simulink model "Bebop5_like3_but_dist_toward_end"  (R2018a)
settings: Solver=VariableStepAuto  StartTime=0.0  StopTime=50  FixedStep=.04  MaxStep=1.00  MinStep=0.005  RelTol=10  AbsTol=10
values from neighbouring files (symbols this model uses):
  flightplan = [dist,0,height,deg2rad(090) ... (first row only)    [compare_cubic_spline_1.m]    (also in initialize_race_realtime.m; initialize_race_realtime_backup_cubic.m; plot_sim.m = [ 4.348, -0.278, height, deg2rad(  0); test_b_spline.m)
  FOV = 1.05    [initialize_race_realtime.m]    (also in initialize_race_realtime_backup_cubic.m)
  g = 9.81    [initialize_race_no_realtime.m]    (also in initialize_race_realtime.m; initialize_race_realtime_backup_cubic.m; moving_average_rls_own.m = P(i-1)*meas*(lambda+meas*P(i-1)*meas)^-1)
  gate_size = 1.4    [initialize_race_realtime.m]    (also in initialize_race_realtime_backup_cubic.m)
  gates = sim_gates(:,:,1)    [eval_sim.m]    (also in initialize_race_realtime.m = [dist,0,height,deg2rad(110); initialize_race_realtime_backup_cubic.m = [dist,0,height,deg2rad(110); plot_sim.m)
  I = [1 0 0 ... (first row only)    [Bebop_sim_init.m]    (also in initialize_race_no_realtime.m; initialize_race_realtime.m; initialize_race_realtime_backup_cubic.m; moving_averge_rls_download.m = ones(1,N))
  init_std_dev = [1.0*ones(1,3),deg2rad(30)]    [initialize_race_realtime.m]    (also in initialize_race_realtime_backup_cubic.m)
  m = 0.68    [calc_plot_spline.m]    (also in calc_spline.m; compare_cubic_spline_1.m = vpasolve(e,r); compare_cubic_spline_2.m = r/3*(-sin(dp)+sqrt(sin(dp)^2-6*cos(dp)+6)); initialize_race_no_realtime.m = 2)
  max_rot_Z = (90)*pi/180    (= 1.57079632679)    [Bebop_sim_init.m]    (also in initialize_race_no_realtime.m = 1.0471975512; initialize_race_realtime.m; initialize_race_realtime_backup_cubic.m; run_batch1.m = list_agility(idx_agility)*max_rot_Z)
  max_theta_X = (40)*pi/180    (= 0.698131700798)    [Bebop_sim_init.m]    (also in initialize_race_no_realtime.m = 0.13962634016; initialize_race_realtime.m = 1.308996939; initialize_race_realtime_backup_cubic.m = 1.308996939; run_batch1.m = list_agility(idx_agility)*max_theta_X)
  max_theta_Y = (40)*pi/180    (= 0.698131700798)    [Bebop_sim_init.m]    (also in initialize_race_no_realtime.m = 0.13962634016; initialize_race_realtime.m = 1.308996939; initialize_race_realtime_backup_cubic.m = 1.308996939; run_batch1.m = list_agility(idx_agility)*max_theta_Y)
  max_v_Z = .5    (= 0.5)    [Bebop_sim_init.m]    (also in initialize_race_no_realtime.m = 1; initialize_race_realtime.m = 3; initialize_race_realtime_backup_cubic.m = 3; run_batch1.m = list_agility(idx_agility)*max_v_Z)
  max_vel = 1.5    [initialize_race_realtime.m]    (also in initialize_race_realtime_backup_cubic.m; run_batch1.m = list_speed(idx_speed); run_batch2.m = list_speed(idx_speed); run_batch3.m = list_speed(idx_speed))
  std_dev_factor = 1.0    (= 1)    [initialize_race_realtime.m]
  std_dev_switch = std_dev_factor/5    (= 0.2)    [initialize_race_realtime.m]
undefined symbols (not defined in the file or in its folder): fspecial, gray, Rec, SDTV
libraries: simulink x11, sharedtransform x11, visionanalysis x7, visiontextngfix x5, visiontransforms x3, aerolibactuator x2, aerolibutil x2, vrlib x2, visionstatistics x2, visionconversions x2, shared6dof x1, visionsinks x1
(part 3 of 4)

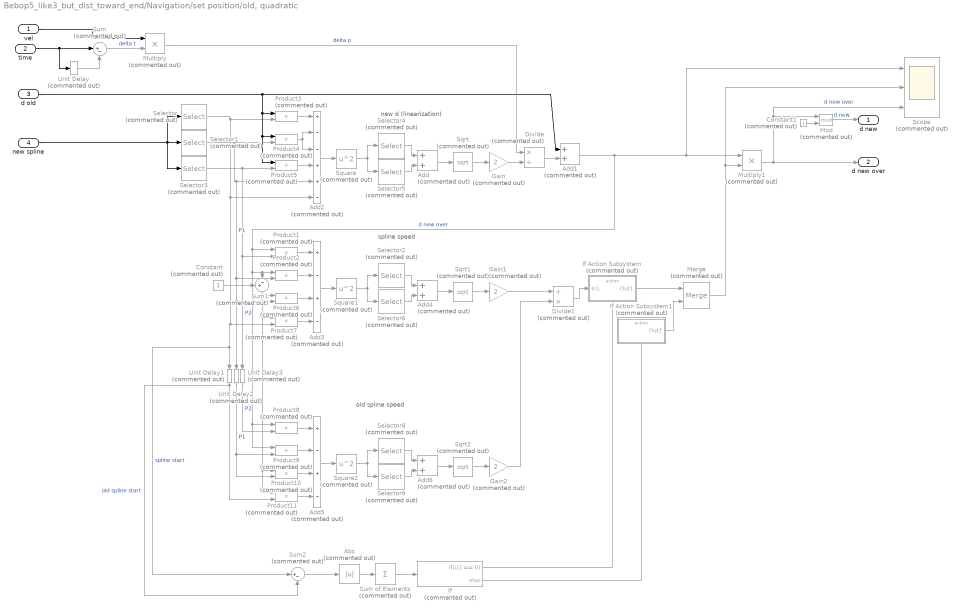
== system Bebop5_like3_but_dist_toward_end/Navigation/set position/old, quadratic ==
  note: old spline speed
  note: spline speed
  note: new d (linearization)
  vel : Inport
  time : Inport  Port=2
  d old : Inport  Port=3
  new spline : Inport  Port=4
  Abs : Abs  Commented=on
  Add{,1,4,6} (4 alike) : Sum  Commented=on
  Add2 : Sum  Commented=on  Inputs=+--++-
  Add3 : Sum  Commented=on  Inputs=+-+-
  Add5 : Sum  Commented=on  Inputs=+-+-
  Constant : Constant  Commented=on
  Constant1 : Constant  Commented=on
  Divide : Product  Commented=on  Inputs=*/
  Divide1 : Product  Commented=on  Inputs=/*
  Gain : Gain  Commented=on  Gain=2
  Gain1 : Gain  Commented=on  Gain=2
  Gain2 : Gain  Commented=on  Gain=2
  If : If  Commented=on  IfExpression=u1 == 0
  If Action Subsystem : Subsystem  Commented=on  TreatAsAtomicUnit=on
  If Action Subsystem1 : Subsystem  Commented=on  TreatAsAtomicUnit=on
  Merge : Merge  Commented=on
  Mod : Math  Commented=on  Operator=mod  SaturateOnIntegerOverflow=on
  Multiply : Product  Commented=on
  Multiply1 : Product  Commented=on
  Product{1..11} (11 alike) : Product  Commented=on
  Scope : Scope  Commented=on  NumInputPorts=3
  Selector : Selector  Commented=on  NumberOfDimensions=2  IndexMode=Zero-based  InputPortWidth=3  IndexOptions=Index vector (dialog),Index vector (dialog)  Indices=0,[0 1 2]  OutputSizes=1,1
  Selector1 : Selector  Commented=on  NumberOfDimensions=2  IndexMode=Zero-based  InputPortWidth=3  IndexOptions=Index vector (dialog),Index vector (dialog)  Indices=1,[0 1 2]  OutputSizes=1,1
  Selector2 : Selector  Commented=on  IndexMode=Zero-based  InputPortWidth=3  IndexOptions=Index vector (dialog)  Indices=1  OutputSizes=1
  Selector3 : Selector  Commented=on  NumberOfDimensions=2  IndexMode=Zero-based  InputPortWidth=3  IndexOptions=Index vector (dialog),Index vector (dialog)  Indices=2,[0 1 2]  OutputSizes=1,1
  Selector4 : Selector  Commented=on  IndexMode=Zero-based  InputPortWidth=3  IndexOptions=Index vector (dialog)  Indices=1  OutputSizes=1
  Selector5 : Selector  Commented=on  IndexMode=Zero-based  InputPortWidth=3  IndexOptions=Index vector (dialog)  Indices=0  OutputSizes=1
  Selector6 : Selector  Commented=on  IndexMode=Zero-based  InputPortWidth=3  IndexOptions=Index vector (dialog)  Indices=0  OutputSizes=1
  Selector8 : Selector  Commented=on  IndexMode=Zero-based  InputPortWidth=3  IndexOptions=Index vector (dialog)  Indices=1  OutputSizes=1
  Selector9 : Selector  Commented=on  IndexMode=Zero-based  InputPortWidth=3  IndexOptions=Index vector (dialog)  Indices=0  OutputSizes=1
  Sqrt : Sqrt  Commented=on  SaturateOnIntegerOverflow=on
  Sqrt1 : Sqrt  Commented=on  SaturateOnIntegerOverflow=on
  Sqrt2 : Sqrt  Commented=on  SaturateOnIntegerOverflow=on
  Square : Math  Commented=on  Operator=square  SaturateOnIntegerOverflow=on
  Square1 : Math  Commented=on  Operator=square  SaturateOnIntegerOverflow=on
  Square2 : Math  Commented=on  Operator=square  SaturateOnIntegerOverflow=on
  Sum : Sum  Commented=on  Inputs=|+-
  Sum of Elements : Sum  Commented=on  Inputs=+
  Sum1 : Sum  Commented=on  Inputs=+-|
  Sum2 : Sum  Commented=on  Inputs=|+-
  Unit Delay{,1..3} (4 alike) : UnitDelay  Commented=on  SampleTime=-1
  d new : Outport
  d new over : Outport  Port=2
  wires:
  Product6/1 -> Add3/3
  Add5/1 -> Square2/1
  If Action Subsystem/1(Out1) -> Merge/1
  Gain/1 -> Divide/2
  Product10/1 -> Add5/3
  Add3/1 -> Square1/1
  Product11/1 -> Add5/4
  Product8/1 -> Add5/1
  Abs/1 -> Sum of Elements/1
  Sum2/1 -> Abs/1
  Gain1/1 -> Divide1/1
  Add4/1 -> Sqrt1/1
  Add1/1 -> Product1/1, Product8/1, Product9/1, Product2/1, Sum1/2, Scope/1, Multiply1/1  "d new over"
  Add/1 -> Sqrt/1
  Product5/1 -> Add2/4
  Selector/1 -> Product3/2, Add2/6, Unit Delay1/1, Sum2/1, Product7/2  "spline start"
  Constant/1 -> Sum1/1
  Sqrt2/1 -> Gain2/1
  Product4/1 -> Add2/2, Add2/3
  Square/1 -> Selector5/1, Selector4/1
  Product2/1 -> Add3/2
  Selector5/1 -> Add/2
  vel/1 -> Multiply/1
  Product3/1 -> Add2/1
  d old/1 -> Add1/1, Product3/1, Product4/1, Product5/1
  Add6/1 -> Sqrt2/1
  Sum1/1 -> Product11/1, Product10/1, Product7/1, Product6/1
  Unit Delay/1 -> Sum/2
  Divide/1 -> Add1/2
  Mod/1 -> d new/1  "d new"
  time/1 -> Unit Delay/1, Sum/1
  Merge/1 -> Scope/2, Multiply1/2
  If/1 -> If Action Subsystem/Action
  Square1/1 -> Selector2/1, Selector6/1
  Selector3/1 -> Product5/2, Unit Delay3/1, Product1/2  "P2"
  new spline/1 -> Selector/1, Selector3/1, Selector1/1
  Selector6/1 -> Add4/2
  Selector1/1 -> Product4/2, Add2/5, Product2/2, Unit Delay2/1, Product6/2  "P1"
  Multiply1/1 -> d new over/1, Scope/3, Mod/1  "d new over"
  Divide1/1 -> If Action Subsystem/1(In1)
  If/2 -> If Action Subsystem1/Action
  Sqrt/1 -> Gain/1
  Product1/1 -> Add3/1
  Unit Delay2/1 -> Product9/2, Product10/2  "P1"
  Add2/1 -> Square/1
  Unit Delay1/1 -> Product11/2, Sum2/2  "old spline start"
  Selector8/1 -> Add6/1
  Sum/1 -> Multiply/2  "delta t"
  Selector9/1 -> Add6/2
  If Action Subsystem1/1(Out1) -> Merge/2
  Sqrt1/1 -> Gain1/1
  Selector2/1 -> Add4/1
  Unit Delay3/1 -> Product8/2  "P2"
  Square2/1 -> Selector8/1, Selector9/1
  Multiply/1 -> Divide/1  "delta p"
  Constant1/1 -> Mod/2
  Product9/1 -> Add5/2
  Sum of Elements/1 -> If/1
  Product7/1 -> Add3/4
  Selector4/1 -> Add/1
  Gain2/1 -> Divide1/2

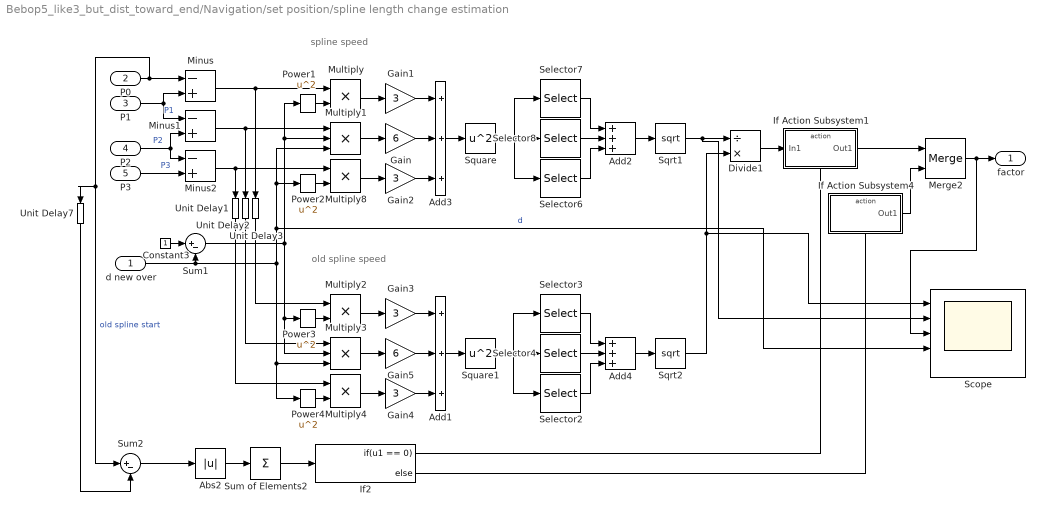
== system Bebop5_like3_but_dist_toward_end/Navigation/set position/spline length change estimation ==
  note: old spline speed
  note: spline speed
  d new over : Inport
  P0 : Inport  Port=2
  P1 : Inport  Port=3
  P2 : Inport  Port=4
  P3 : Inport  Port=5
  Abs2 : Abs
  Add{1..4} (4 alike) : Sum  Inputs=+++
  Constant3 : Constant
  Divide1 : Product  Inputs=/*
  Gain : Gain  Gain=6
  Gain{1..4} (4 alike) : Gain  Gain=3
  Gain5 : Gain  Gain=6
  If Action Subsystem1 : Subsystem  TreatAsAtomicUnit=on
  If Action Subsystem4 : Subsystem  TreatAsAtomicUnit=on
  If2 : If  IfExpression=u1 == 0
  Merge2 : Merge
  Minus : Sum  Inputs=-+
  Minus1 : Sum  Inputs=-+
  Minus2 : Sum  Inputs=-+
  Multiply{,2,4,8} (4 alike) : Product
  Multiply1 : Product  Inputs=3
  Multiply3 : Product  Inputs=3
  Power{1..4} (4 alike) : Math  Operator=square  SaturateOnIntegerOverflow=on
  Scope : Scope  NumInputPorts=5
  Selector2 : Selector  IndexMode=Zero-based  InputPortWidth=3  IndexOptions=Index vector (dialog)  Indices=2  OutputSizes=1
  Selector3 : Selector  IndexMode=Zero-based  InputPortWidth=3  IndexOptions=Index vector (dialog)  Indices=0  OutputSizes=1
  Selector4 : Selector  IndexMode=Zero-based  InputPortWidth=3  IndexOptions=Index vector (dialog)  Indices=1  OutputSizes=1
  Selector6 : Selector  IndexMode=Zero-based  InputPortWidth=3  IndexOptions=Index vector (dialog)  Indices=2  OutputSizes=1
  Selector7 : Selector  IndexMode=Zero-based  InputPortWidth=3  IndexOptions=Index vector (dialog)  Indices=0  OutputSizes=1
  Selector8 : Selector  IndexMode=Zero-based  InputPortWidth=3  IndexOptions=Index vector (dialog)  Indices=1  OutputSizes=1
  Sqrt1 : Sqrt  SaturateOnIntegerOverflow=on
  Sqrt2 : Sqrt  SaturateOnIntegerOverflow=on
  Square : Math  Operator=square  SaturateOnIntegerOverflow=on
  Square1 : Math  Operator=square  SaturateOnIntegerOverflow=on
  Sum of Elements2 : Sum  Inputs=+
  Sum1 : Sum  Inputs=|+-
  Sum2 : Sum  Inputs=|+-
  Unit Delay{1..3,7} (4 alike) : UnitDelay  SampleTime=-1
  factor : Outport
  wires:
  P2/1 -> Minus1/2, Minus2/1  "P2"
  Power1/1 -> Multiply/2
  Minus1/1 -> Unit Delay2/1, Multiply1/1
  Constant3/1 -> Sum1/1
  Minus/1 -> Unit Delay3/1, Multiply/1
  P1/1 -> Minus/2, Minus1/1  "P1"
  Multiply8/1 -> Gain2/1
  Power2/1 -> Multiply8/2
  Multiply/1 -> Gain1/1
  P3/1 -> Minus2/2  "P3"
  Minus2/1 -> Unit Delay1/1, Multiply8/1
  Multiply1/1 -> Gain/1
  Gain/1 -> Add3/2
  Power3/1 -> Multiply2/2
  Multiply2/1 -> Gain3/1
  Gain5/1 -> Add1/2
  Multiply4/1 -> Gain4/1
  Power4/1 -> Multiply4/2
  Multiply3/1 -> Gain5/1
  Unit Delay1/1 -> Multiply4/1
  d new over/1 -> Sum1/2, Power4/1, Multiply3/3, Scope/4, Multiply1/3, Power2/1  "d"
  Unit Delay3/1 -> Multiply2/1
  Unit Delay2/1 -> Multiply3/1
  Sum1/1 -> Multiply3/2, Power3/1, Power1/1, Multiply1/2
  Selector7/1 -> Add2/1
  Selector6/1 -> Add2/3
  Add2/1 -> Sqrt1/1
  Selector8/1 -> Add2/2
  Selector4/1 -> Add4/2
  Selector3/1 -> Add4/1
  Selector2/1 -> Add4/3
  Add4/1 -> Sqrt2/1
  Add3/1 -> Square/1
  Add1/1 -> Square1/1
  Abs2/1 -> Sum of Elements2/1
  Sum of Elements2/1 -> If2/1
  Sum2/1 -> Abs2/1
  Unit Delay7/1 -> Sum2/2
  P0/1 -> Sum2/1, Unit Delay7/1, Minus/1  "old spline start"
  If2/1 -> If Action Subsystem1/Action
  Sqrt2/1 -> Scope/1, Divide1/2
  Sqrt1/1 -> Scope/2, Divide1/1
  If2/2 -> If Action Subsystem4/Action
  If Action Subsystem1/1(Out1) -> Merge2/1
  Divide1/1 -> If Action Subsystem1/1(In1)
  If Action Subsystem4/1(Out1) -> Merge2/2
  Merge2/1 -> Scope/3, factor/1
  Gain1/1 -> Add3/1
  Gain2/1 -> Add3/3
  Gain3/1 -> Add1/1
  Gain4/1 -> Add1/3
  Square/1 -> Selector6/1, Selector7/1, Selector8/1
  Square1/1 -> Selector2/1, Selector3/1, Selector4/1

== system Bebop5_like3_but_dist_toward_end/Vision System/Harris corner detection/Harris Corners ==
  Threshold : Inport
  Corner Detection : visionanalysis/Corner Detection  method=Harris corner detection (Harris & Stephens)  factor=0.01  filter=fspecial('gaussian', [1 9], 3)  thrInten=0.1  thrAngle=157.5  output=Obsolete9b  outputInUse=Corner location  maxNum=5  thrMetric=0.01  neighborSize=[25 25]  isOutVarDim=on  accumMode=Binary point scaling  accumWordLength=32  accumFracLength=0  prodOutputMode=Binary point scaling  prodOutputWordLength=32  prodOutputFracLength=0  memoryMode=Binary point scaling  memoryWordLength=32  memoryFracLength=0  firstCoeffMode=Specify word length  firstCoeffWordLength=16  firstCoeffFracLength=17  roundingMode=Floor  overflowMode=off
      settings: SourceProductName=Computer Vision System Toolbox  SourceProductBaseCode=VP
  Gaussian Pyramid : visiontransforms/Gaussian Pyramid  Commented=on  operation=Expand  level=1  source=Specify via dialog  a=0.375  coef=fspecial('gaussian', [1 9], 3)  hiddenCoef=fspecial('gaussian', [1 9], 3)  firstCoeffMode=Specify word length  firstCoeffWordLength=16  firstCoeffFracLength=17  outputMode=Binary point scaling  outputWordLength=32  outputFracLength=10  prodOutputMode=Binary point scaling  prodOutputWordLength=32  prodOutputFracLength=10  roundingMode=Floor  overflowMode=off
      settings: SourceProductName=Computer Vision System Toolbox  SourceProductBaseCode=VP
  Video Viewer2 : VideoViewer  Commented=on  colormapValue=gray(256)  FigPos=[76 898 768 763]
  Corners : Outport
  wires:
  Threshold/1 -> Gaussian Pyramid/1, Corner Detection/1
  Gaussian Pyramid/1 -> Video Viewer2/1
  Corner Detection/1 -> Corners/1

== system Bebop5_like3_but_dist_toward_end/Vision System/Harris corner detection/calculate corners ==
  In1 : Inport
  Action Port : ActionPort  PropagateVarSize=During execution  ActionType=then
  calculate corners : MATLAB Function  TreatAsAtomicUnit=on
  Out1 : Outport
  wires:
  In1/1 -> calculate corners/1(corners)
  calculate corners/1(corners_four) -> Out1/1

== system Bebop5_like3_but_dist_toward_end/Control/Control algorithm/Create Path Frame/Make X Vector ==
  Velocity Vector : Inport
  Make Unit : Subsystem
  X Vector : Outport
  wires:
  Velocity Vector/1 -> Make Unit/1(Vector)
  Make Unit/1(Unit Vector) -> X Vector/1

== system Bebop5_like3_but_dist_toward_end/Control/Control algorithm/Create Path Frame/Make Y Vector ==
  Velocity Vector : Inport
  Constant : Constant  Value=0
  Demux : Demux  Outputs=3
  Gain : Gain  Gain=-1
  Make Unit : Subsystem
  Matrix Concatenate : Concatenate  NumInputs=3  Mode=Multidimensional array
  Terminator : Terminator
  Y Vector : Outport
  wires:
  Make Unit/1(Unit Vector) -> Y Vector/1
  Velocity Vector/1 -> Demux/1
  Demux/3 -> Terminator/1
  Demux/2 -> Gain/1
  Gain/1 -> Matrix Concatenate/1
  Demux/1 -> Matrix Concatenate/2
  Constant/1 -> Matrix Concatenate/3
  Matrix Concatenate/1 -> Make Unit/1(Vector)

== system Bebop5_like3_but_dist_toward_end/Control/Control algorithm/Create Path Frame/Make Z Vector ==
  Velocity Vector : Inport
  Add : Sum
  Demux : Demux  Outputs=3
  Gain : Gain  Gain=-1
  Gain1 : Gain  Gain=-1
  Make Unit : Subsystem
  Matrix Concatenate : Concatenate  NumInputs=3  Mode=Multidimensional array
  Multiply : Product
  Multiply1 : Product
  Square : Math  Operator=square  SaturateOnIntegerOverflow=on
  Square1 : Math  Operator=square  SaturateOnIntegerOverflow=on
  Z Vector : Outport
  wires:
  Make Unit/1(Unit Vector) -> Z Vector/1
  Velocity Vector/1 -> Demux/1
  Demux/3 -> Multiply/2, Multiply1/2
  Matrix Concatenate/1 -> Make Unit/1(Vector)
  Multiply/1 -> Gain/1
  Gain/1 -> Matrix Concatenate/1
  Demux/1 -> Square/1, Multiply/1
  Multiply1/1 -> Gain1/1
  Gain1/1 -> Matrix Concatenate/2
  Demux/2 -> Square1/1, Multiply1/1
  Add/1 -> Matrix Concatenate/3
  Square/1 -> Add/1
  Square1/1 -> Add/2

== system Bebop5_like3_but_dist_toward_end/Navigation/calc v/Create Path Frame/Make X Vector ==
  Velocity Vector : Inport
  Make Unit : Subsystem
  Transpose : Math  Operator=transpose  SaturateOnIntegerOverflow=on
  X Vector : Outport
  wires:
  Velocity Vector/1 -> Make Unit/1(Vector)
  Make Unit/1(Unit Vector) -> Transpose/1
  Transpose/1 -> X Vector/1

== system Bebop5_like3_but_dist_toward_end/Navigation/calc v/Create Path Frame/Make Y Vector ==
  Velocity Vector : Inport
  Constant : Constant  Value=0
  Demux : Demux  Outputs=3
  Gain : Gain  Gain=-1
  Make Unit : Subsystem
  Matrix Concatenate : Concatenate  NumInputs=3  Mode=Multidimensional array
  Terminator : Terminator
  Y Vector : Outport
  wires:
  Make Unit/1(Unit Vector) -> Y Vector/1
  Velocity Vector/1 -> Demux/1
  Demux/3 -> Terminator/1
  Demux/2 -> Gain/1
  Gain/1 -> Matrix Concatenate/1
  Demux/1 -> Matrix Concatenate/2
  Constant/1 -> Matrix Concatenate/3
  Matrix Concatenate/1 -> Make Unit/1(Vector)

== system Bebop5_like3_but_dist_toward_end/Navigation/calc v/Create Path Frame/Make Z Vector ==
  Velocity Vector : Inport
  Add : Sum
  Demux : Demux  Outputs=3
  Gain : Gain  Gain=-1
  Gain1 : Gain  Gain=-1
  Make Unit : Subsystem
  Matrix Concatenate : Concatenate  NumInputs=3  Mode=Multidimensional array
  Multiply : Product
  Multiply1 : Product
  Square : Math  Operator=square  SaturateOnIntegerOverflow=on
  Square1 : Math  Operator=square  SaturateOnIntegerOverflow=on
  Z Vector : Outport
  wires:
  Make Unit/1(Unit Vector) -> Z Vector/1
  Velocity Vector/1 -> Demux/1
  Demux/3 -> Multiply/2, Multiply1/2
  Matrix Concatenate/1 -> Make Unit/1(Vector)
  Multiply/1 -> Gain/1
  Gain/1 -> Matrix Concatenate/1
  Demux/1 -> Square/1, Multiply/1
  Multiply1/1 -> Gain1/1
  Gain1/1 -> Matrix Concatenate/2
  Demux/2 -> Square1/1, Multiply1/1
  Add/1 -> Matrix Concatenate/3
  Square/1 -> Add/1
  Square1/1 -> Add/2

== system Bebop5_like3_but_dist_toward_end/Navigation/calc v/calculate direction B'(d)/old, quadratic ==
  note: B'(d) = 2(1-d)(P1-P0) + 2d(P2-P1) = 2*(dP0-2dP1+dP2+P1-P0)
  d : Inport
  P0 : Inport  Port=2
  P1 : Inport  Port=3
  P2 : Inport  Port=4
  vel : Inport  Port=5
  Add1 : Sum  Commented=on  Inputs=+--++-
  Atan1 : Trigonometry  Commented=on  Operator=atan2
  Constant1 : Constant  Commented=on  Value=0
  Constant2 : Constant  Commented=on  Value=0
  Matrix Multiply : Product  Commented=on  Inputs=/*  Multiplication=Matrix(*)
  Product : Product  Commented=on
  Product1 : Product  Commented=on
  Product2 : Product  Commented=on
  Rotation Angles to Direction Cosine Matrix1 : sharedtransform/Rotation Angles to Direction Cosine Matrix  Commented=on  rotationOrder=ZYX  aMode=aMode
      settings: SourceProductBaseCode=AE
  Selector7 : Selector  Commented=on  IndexMode=Zero-based  InputPortWidth=3  IndexOptions=Index vector (dialog)  Indices=1  OutputSizes=1
  Selector8 : Selector  Commented=on  IndexMode=Zero-based  InputPortWidth=3  IndexOptions=Index vector (dialog)  Indices=0  OutputSizes=1
  Vector Concatenate : Concatenate  Commented=on  NumInputs=3
  Vector Concatenate1 : Concatenate  Commented=on  NumInputs=3
  Out1 : Outport
  wires:
  Product2/1 -> Add1/4
  P1/1 -> Add1/5, Product1/2
  Rotation Angles to Direction Cosine Matrix1/1 -> Matrix Multiply/1  "rot matrix"
  P2/1 -> Product2/2
  Add1/1 -> Selector8/1, Selector7/1
  Product/1 -> Add1/1
  P0/1 -> Add1/6, Product/2
  d/1 -> Product2/1, Product1/1, Product/1
  Constant1/1 -> Vector Concatenate/2, Vector Concatenate/3
  Vector Concatenate1/1 -> Matrix Multiply/2
  Product1/1 -> Add1/3, Add1/2
  Vector Concatenate/1 -> Rotation Angles to Direction Cosine Matrix1/1
  Selector7/1 -> Atan1/1
  vel/1 -> Vector Concatenate1/1
  Constant2/1 -> Vector Concatenate1/2, Vector Concatenate1/3
  Matrix Multiply/1 -> Out1/1
  Selector8/1 -> Atan1/2
  Atan1/1 -> Vector Concatenate/1  "yaw"

== system Bebop5_like3_but_dist_toward_end/Navigation/calculate desired/calc pos B(d)/old, quadratic ==
  note: B(d) = (1-d)*u.*((1-d)*P0+d*P1)+d*u.*((1-d)*P1 + d*P2);
  d : Inport
  In2 : Inport  Port=2
  In3 : Inport  Port=3
  In4 : Inport  Port=4
  Add : Sum  Commented=on
  Add1 : Sum  Commented=on
  Add2 : Sum  Commented=on
  Constant : Constant  Commented=on
  Multiply{2..7} (6 alike) : Product  Commented=on
  Sum : Sum  Commented=on  Inputs=|+-
  Out1 : Outport
  wires:
  In4/1 -> Multiply5/1
  Constant/1 -> Sum/1
  Multiply7/1 -> Add2/2
  d/1 -> Multiply5/2, Multiply7/1, Multiply3/1, Sum/2
  Multiply3/1 -> Add/2
  Multiply5/1 -> Add1/2
  Multiply4/1 -> Add1/1
  Sum/1 -> Multiply4/2, Multiply6/2, Multiply2/1  "1-d"
  In3/1 -> Multiply4/1, Multiply3/2
  Multiply2/1 -> Add/1
  Add2/1 -> Out1/1
  Add1/1 -> Multiply7/2
  Multiply6/1 -> Add2/1
  In2/1 -> Multiply2/2
  Add/1 -> Multiply6/1

== system Bebop5_like3_but_dist_toward_end/Navigation/calculate desired/calculate direction B'(d)/Make Unit ==
  Vector : Inport
  Multiply : Product
  Reciprocal Sqrt : Sqrt  Operator=rSqrt  SaturateOnIntegerOverflow=on
  Square : Math  Operator=square  SaturateOnIntegerOverflow=on
  Sum of Elements : Sum  Inputs=+
  Transpose : Math  Operator=transpose  SaturateOnIntegerOverflow=on
  Unit Vector : Outport
  wires:
  Reciprocal Sqrt/1 -> Multiply/1
  Vector/1 -> Square/1, Multiply/2
  Square/1 -> Sum of Elements/1
  Multiply/1 -> Transpose/1
  Sum of Elements/1 -> Reciprocal Sqrt/1
  Transpose/1 -> Unit Vector/1

== system Bebop5_like3_but_dist_toward_end/Navigation/calculate desired/calculate direction B'(d)/old, quadratic ==
  note: B'(d) = 2(1-d)(P1-P0) + 2d(P2-P1) = 2*(dP0-2dP1+dP2+P1-P0)
  d : Inport
  P0 : Inport  Port=2
  P1 : Inport  Port=3
  P2 : Inport  Port=4
  vel : Inport  Port=5
  Add1 : Sum  Commented=on  Inputs=+--++-
  Atan1 : Trigonometry  Commented=on  Operator=atan2
  Constant1 : Constant  Commented=on  Value=0
  Constant2 : Constant  Commented=on  Value=0
  Matrix Multiply : Product  Commented=on  Inputs=/*  Multiplication=Matrix(*)
  Product : Product  Commented=on
  Product1 : Product  Commented=on
  Product2 : Product  Commented=on
  Rotation Angles to Direction Cosine Matrix1 : sharedtransform/Rotation Angles to Direction Cosine Matrix  Commented=on  rotationOrder=ZYX  aMode=aMode
      settings: SourceProductBaseCode=AE
  Selector7 : Selector  Commented=on  IndexMode=Zero-based  InputPortWidth=3  IndexOptions=Index vector (dialog)  Indices=1  OutputSizes=1
  Selector8 : Selector  Commented=on  IndexMode=Zero-based  InputPortWidth=3  IndexOptions=Index vector (dialog)  Indices=0  OutputSizes=1
  Vector Concatenate : Concatenate  Commented=on  NumInputs=3
  Vector Concatenate1 : Concatenate  Commented=on  NumInputs=3
  Out1 : Outport
  wires:
  Product2/1 -> Add1/4
  P1/1 -> Add1/5, Product1/2
  Rotation Angles to Direction Cosine Matrix1/1 -> Matrix Multiply/1  "rot matrix"
  P2/1 -> Product2/2
  Add1/1 -> Selector8/1, Selector7/1
  Product/1 -> Add1/1
  P0/1 -> Add1/6, Product/2
  d/1 -> Product2/1, Product1/1, Product/1
  Constant1/1 -> Vector Concatenate/2, Vector Concatenate/3
  Vector Concatenate1/1 -> Matrix Multiply/2
  Product1/1 -> Add1/3, Add1/2
  Vector Concatenate/1 -> Rotation Angles to Direction Cosine Matrix1/1
  Selector7/1 -> Atan1/1
  vel/1 -> Vector Concatenate1/1
  Constant2/1 -> Vector Concatenate1/2, Vector Concatenate1/3
  Matrix Multiply/1 -> Out1/1
  Selector8/1 -> Atan1/2
  Atan1/1 -> Vector Concatenate/1  "yaw"

== system Bebop5_like3_but_dist_toward_end/Navigation/set position/old, quadratic/If Action Subsystem ==
  In1 : Inport
  Action Port : ActionPort  ActionType=then
  Out1 : Outport
  wires:
  In1/1 -> Out1/1

== system Bebop5_like3_but_dist_toward_end/Navigation/set position/old, quadratic/If Action Subsystem1 ==
  Action Port : ActionPort  ActionType=else
  Constant : Constant
  Out1 : Outport
  wires:
  Constant/1 -> Out1/1

== system Bebop5_like3_but_dist_toward_end/Navigation/set position/spline length change estimation/If Action Subsystem1 ==
  In1 : Inport
  Action Port : ActionPort  ActionType=then
  Out1 : Outport
  wires:
  In1/1 -> Out1/1

== system Bebop5_like3_but_dist_toward_end/Navigation/set position/spline length change estimation/If Action Subsystem4 ==
  Action Port : ActionPort  ActionType=else
  Constant : Constant
  Out1 : Outport
  wires:
  Constant/1 -> Out1/1

== system Bebop5_like3_but_dist_toward_end/Control/Control algorithm/Create Path Frame/Make X Vector/Make Unit ==
  Vector : Inport
  Multiply : Product
  Reciprocal Sqrt : Sqrt  Operator=rSqrt  SaturateOnIntegerOverflow=on
  Square : Math  Operator=square  SaturateOnIntegerOverflow=on
  Sum of Elements : Sum  Inputs=+
  Unit Vector : Outport
  wires:
  Reciprocal Sqrt/1 -> Multiply/1
  Vector/1 -> Square/1, Multiply/2
  Square/1 -> Sum of Elements/1
  Multiply/1 -> Unit Vector/1
  Sum of Elements/1 -> Reciprocal Sqrt/1

== system Bebop5_like3_but_dist_toward_end/Control/Control algorithm/Create Path Frame/Make Y Vector/Make Unit ==
  Vector : Inport
  Multiply : Product
  Reciprocal Sqrt : Sqrt  Operator=rSqrt  SaturateOnIntegerOverflow=on
  Square : Math  Operator=square  SaturateOnIntegerOverflow=on
  Sum of Elements : Sum  Inputs=+
  Unit Vector : Outport
  wires:
  Reciprocal Sqrt/1 -> Multiply/1
  Vector/1 -> Square/1, Multiply/2
  Square/1 -> Sum of Elements/1
  Multiply/1 -> Unit Vector/1
  Sum of Elements/1 -> Reciprocal Sqrt/1

== system Bebop5_like3_but_dist_toward_end/Control/Control algorithm/Create Path Frame/Make Z Vector/Make Unit ==
  Vector : Inport
  Multiply : Product
  Reciprocal Sqrt : Sqrt  Operator=rSqrt  SaturateOnIntegerOverflow=on
  Square : Math  Operator=square  SaturateOnIntegerOverflow=on
  Sum of Elements : Sum  Inputs=+
  Unit Vector : Outport
  wires:
  Reciprocal Sqrt/1 -> Multiply/1
  Vector/1 -> Square/1, Multiply/2
  Square/1 -> Sum of Elements/1
  Multiply/1 -> Unit Vector/1
  Sum of Elements/1 -> Reciprocal Sqrt/1

== system Bebop5_like3_but_dist_toward_end/Navigation/calc v/Create Path Frame/Make X Vector/Make Unit ==
  Vector : Inport
  Multiply : Product
  Reciprocal Sqrt : Sqrt  Operator=rSqrt  SaturateOnIntegerOverflow=on
  Square : Math  Operator=square  SaturateOnIntegerOverflow=on
  Sum of Elements : Sum  Inputs=+
  Unit Vector : Outport
  wires:
  Reciprocal Sqrt/1 -> Multiply/1
  Vector/1 -> Square/1, Multiply/2
  Square/1 -> Sum of Elements/1
  Multiply/1 -> Unit Vector/1
  Sum of Elements/1 -> Reciprocal Sqrt/1

== system Bebop5_like3_but_dist_toward_end/Navigation/calc v/Create Path Frame/Make Y Vector/Make Unit ==
  Vector : Inport
  Multiply : Product
  Reciprocal Sqrt : Sqrt  Operator=rSqrt  SaturateOnIntegerOverflow=on
  Square : Math  Operator=square  SaturateOnIntegerOverflow=on
  Sum of Elements : Sum  Inputs=+
  Unit Vector : Outport
  wires:
  Reciprocal Sqrt/1 -> Multiply/1
  Vector/1 -> Square/1, Multiply/2
  Square/1 -> Sum of Elements/1
  Multiply/1 -> Unit Vector/1
  Sum of Elements/1 -> Reciprocal Sqrt/1

== system Bebop5_like3_but_dist_toward_end/Navigation/calc v/Create Path Frame/Make Z Vector/Make Unit ==
  Vector : Inport
  Multiply : Product
  Reciprocal Sqrt : Sqrt  Operator=rSqrt  SaturateOnIntegerOverflow=on
  Square : Math  Operator=square  SaturateOnIntegerOverflow=on
  Sum of Elements : Sum  Inputs=+
  Unit Vector : Outport
  wires:
  Reciprocal Sqrt/1 -> Multiply/1
  Vector/1 -> Square/1, Multiply/2
  Square/1 -> Sum of Elements/1
  Multiply/1 -> Unit Vector/1
  Sum of Elements/1 -> Reciprocal Sqrt/1

== matlab function Bebop5_like3_but_dist_toward_end/Vision System/Harris corner detection/calculate corners/calculate corners ==
  data: corners_four output; corners input
function corners_four = calculate_corners(corners)
    
    
    %% get bounding box
    corners = double(corners);
    box=[0,0,0,0];
    box(1) = min(corners(:,1));
    box(2) = max(corners(:,1));
    box(3) = min(corners(:,2));
    box(4) = max(corners(:,2));
    
    corners_box = ([box(1), box(3);
                    box(2), box(3);
                    box(1), box(4);
                    box(2), box(4)]);
                
    corners_four = int32(zeros(4,2));
                
    for m = 1:4
        box = corners_box(m,:);
        multi_box = ones(size(corners,1),1) * box;
        diff = multi_box - corners;
        dist = diff(:,1).^2 + diff(:,2).^2;
        [~,i] = min(dist);
        corners_four(m,:) = corners(i,:);
        corners(i,:)=[];
    end
    
end

== matlab function Bebop5_like3_but_dist_toward_end/Navigation/set position/calculate passed distance ==
  data: d input; spline_new input; d_new output; spline_old input
function d_new = calculate_factor(d,spline_new,spline_old)

    P0_old = spline_old(1,:);
    P1_old = spline_old(2,:);
    P2_old = spline_old(3,:);
    P3_old = spline_old(4,:);
    P0_new = spline_new(1,:);
    P1_new = spline_new(2,:);
    P2_new = spline_new(3,:);
    P3_new = spline_new(4,:);
    
    if ~isequal(P0_old,P0_new)
        d_new = d;
        return
    end
    
    dx0_new=P1_new(1)-P0_new(1);
    dx1_new=P2_new(1)-P1_new(1);
    dx2_new=P3_new(1)-P2_new(1);
    dy0_new=P1_new(2)-P0_new(2);
    dy1_new=P2_new(2)-P1_new(2);
    dy2_new=P3_new(2)-P2_new(2);
    dx0_old=P1_old(1)-P0_old(1);
    dx1_old=P2_old(1)-P1_old(1);
    dx2_old=P3_old(1)-P2_old(1);
    dy0_old=P1_old(2)-P0_old(2);
    dy1_old=P2_old(2)-P1_old(2);
    dy2_old=P3_old(2)-P2_old(2);
    
    fun_new = @(d_s) 3*sqrt((1-d_s).^4*(dx0_new^2+dy0_new^2)+4*d_s.^2.*(1-d_s).^2*(dx1_new^2+dy1_new^2)+d_s.^4*(dx2_new^2+dy2_new^2)+4*d_s.*(1-d_s).^3*(dx0_new*dx1_new+dy0_new*dy1_new)+2*d_s.^2.*(1-d_s).^2*(dx0_new*dx2_new+dy0_new*dy2_new)+4*d_s.^3.*(1-d_s)*(dx1_new*dx2_new+dy1_new*dy2_new));
    fun_old = @(d_s) 3*sqrt((1-d_s).^4*(dx0_old^2+dy0_old^2)+4*d_s.^2.*(1-d_s).^2*(dx1_old^2+dy1_old^2)+d_s.^4*(dx2_old^2+dy2_old^2)+4*d_s.*(1-d_s).^3*(dx0_old*dx1_old+dy0_old*dy1_old)+2*d_s.^2.*(1-d_s).^2*(dx0_old*dx2_old+dy0_old*dy2_old)+4*d_s.^3.*(1-d_s)*(dx1_old*dx2_old+dy1_old*dy2_old));
%     fnc=3*sqrt((1-d_s)^4*(dx0^2+dy0^2)+4*d_s^2*(1-d_s)^2*(dx1^2+dy1^2)+d_s^4*(dx2^2+dy2^2)+4*d_s*(1-d_s)^3*(dx0*dx1+dy0*dy1)+2*d_s^2*(1-d_s)^2*(dx0*dx2+dy0*dy2)+4*d_s^3*(1-d_s)*(dx1*dx2+dy1*dy2));
%     fnc_num = subs(fnc,d_s,d_num);
    
    d_num = 0:0.01:(d-0.01);
    dist_new = 0.01*sum(fun_new(d_num));
    dist_old = 0.01*sum(fun_old(d_num));
    
%     dist_new = integral(fun_new,0,d);
%     dist_old = integral(fun_old,0,d);
    
    d_new = d + (dist_old-dist_new)/fun_new(d);

== matlab function Bebop5_like3_but_dist_toward_end/Initialize/reset_plot ==
function reset_plot()
coder.extrinsic('quiver3')
coder.extrinsic('legend')
close all;
figure('units','normalized','outerposition',[0 0 0.5 1])
hold on
grid on
axis equal

legends=zeros(12,1);
legends(1)=plot3(0,0,-100,'m.','MarkerSize',7);
legends(2)=plot3(0,0,-100,'k.','MarkerSize',5);
legends(3)=quiver3(0,0,-100,0,0,0,0,'c','MaxHeadSize',1,'LineWidth',2);
legends(4)=quiver3(0,0,-100,0,0,0,0,'r','MaxHeadSize',1,'LineWidth',2);
legends(5)=plot3(0,0,-100,':','Color',[1,0.7,0],'LineWidth',2);
legends(6)=plot3(0,0,-100,'kx-','LineWidth',1.2,'MarkerIndices',1,'MarkerSize',10);
legends(7)=plot3(0,0,-100,'r--','LineWidth',1.5);
legends(8)=plot3(0,0,-100,'g--','LineWidth',1.5);
legends(9)=plot3(0,0,-100,'b--','LineWidth',1.5);
legends(10)=plot3(0,0,-100,'b+-','LineWidth',1.2,'MarkerIndices',1,'MarkerSize',10);
legends(11)=quiver3(0,0,-100,0,0,0,0,'b','MaxHeadSize',1,'LineWidth',2);
legends(12)=plot3(0,0,-100,':r','LineWidth',1);
legend(legends(1:12),'flown track','ground track','inactive WP +ori','active WP +ori','spline','drone pos+vel','drone x','drone y','drone z','des pos+vel','measured WP','std dev (x,y,th)','Location','eastoutside','AutoUpdate','off')

for i=1:25
    plot3(0,0,-100,'.')
end

% axis([-5,5,-5,5,-2,2])
axis([-5,5,-5,5,0,4])
% axis([1,4,-2,2,0,4])
%view(-20,40) % 3D view
view(-90,90) % top view
%view(-90,0) % front view
xlabel('x')
ylabel('y')
zlabel('z')

== matlab function Bebop5_like3_but_dist_toward_end/conv/global2strange drone/MATLAB Function ==
  data: euler input; axang_strange output
function axang_strange = fcn(euler)
m1=zeros(3,3);
m1 = eul2rotm([euler(3),euler(2),euler(1)]);
m2 = eul2rotm([-pi/2, 0, pi/2]);

axang_strange = rotm2axang(m1*m2);

== matlab function Bebop5_like3_but_dist_toward_end/Vision System/Harris corner detection/calculate_PnP ==
  data: tVec output; corners input; size input; rMat output
function [tVec, rMat] = calculate_PnP(corners, size)
    tVec=zeros(1,3);
    rMat=zeros(3,3);
    
    Resolution = 1.5*[320, 200];
    vertFOV = 1.05;
    f = 0.5*Resolution(2)/tan(0.5*vertFOV);
    IntrinsicMatrix = [f, 0, 0;
        0, f, 0;
        Resolution/2, 1];
    cameraParams = cameraParameters('IntrinsicMatrix',IntrinsicMatrix); 
    
    %% calculate extrinsics
    worldPoints = size/2*[1 1;
        1 -1;
        -1 1;
        -1 -1];
    
    corners=double(corners);
    if corners == zeros(4,2)
        disp('no corners')
        return
    end
    
    angles = zeros(6,1);
    k = 1;
    for m=1:3
        for n=m+1:4
            angles(k)=atan2(corners(m,2)-corners(n,2),corners(m,1)-corners(n,1));
            k = k+1;            
        end
    end
    
%     angles(angles<=0) = angles(angles<=0)+pi;
%     
%     a = zeros(2,1);
%     a = hist(angles,unique(angles));
%     if max(a)>2
%         disp('three occurences')
%         return
%     end
%     
%     
%     

    % check how much it resembles rectangle
    if abs(max(corners(:,1))-min(corners(:,1))) < 5
        disp('no rectangle 1')
        corners
        return
    elseif abs(max(corners(:,2))-min(corners(:,2))) < 5
        disp('no rectangle 2')
        corners
        return
    end
    
    angles = zeros(2,1);
    angles(1)=atan2(corners(1,2)-corners(4,2),corners(1,1)-corners(4,1));
    angles(2)=atan2(corners(2,2)-corners(3,2),corners(2,1)-corners(3,1));
    angles(angles<=0) = angles(angles<=0)+pi;
    
    if ~(isequal(unique(angles),sort(angles)))
        temp = corners(3,:);
        corners(3,:) = corners(4,:);
        corners(4,:) = temp;
    end
    
    angles(1)=atan2(corners(1,2)-corners(4,2),corners(1,1)-corners(4,1));
    angles(2)=atan2(corners(2,2)-corners(3,2),corners(2,1)-corners(3,1));
    angles(angles<=0) = angles(angles<=0)+pi;
    
    if ~(isequal(unique(angles),sort(angles)))
        disp('still bad after sort')
        corners
        return
    end    
        
    [rMat,tVec] = extrinsics(corners,worldPoints,cameraParams);
%     [orientation,location] = extrinsicsToCameraPose(rMat,tVec);
    
end

== matlab function Bebop5_like3_but_dist_toward_end/Gate info/Yaw2Axang4/MATLAB Function1 ==
  data: axang output; q input
function axang = fcn(q)

axang = zeros(4,1);

angle = 2 * acos(q(1));
x = q(2) / sqrt(1-q(1)*q(1));
y = q(3) / sqrt(1-q(1)*q(1));
z = q(4) / sqrt(1-q(1)*q(1));

if all(isnan([x,y,z]))
    x = 1;
    y = 0;
    z = 0;
end

axang(1) = x;
axang(2) = y;
axang(3) = z;
axang(4) = angle;

== matlab function Bebop5_like3_but_dist_toward_end/conv/global2strange drone/MATLAB Function1 ==
  data: axang output; q input
function axang = fcn(q)

axang = zeros(4,1);

angle = 2 * acos(q(1));
x = q(2) / sqrt(1-q(1)*q(1));
y = q(3) / sqrt(1-q(1)*q(1));
z = q(4) / sqrt(1-q(1)*q(1));

axang(1) = x;
axang(2) = y;
axang(3) = z;
axang(4) = angle;

== matlab function Bebop5_like3_but_dist_toward_end/Plot ==
  data: inbus input
function plot3d(inbus)
%#codegen
coder.extrinsic('delete')
% coder.extrinsic('ellipsoid')
% coder.extrinsic('viscircles')
% coder.extrinsic('quiver3')
% coder.extrinsic('legend')
std_dev_factor = 1.0;

drone_vel = inbus.state.vel;
drone_pos = inbus.state.pos;
drone_ori = inbus.state.eul;
WP_curr_eul = inbus.WP_curr.eul;
WP_curr_pos = inbus.WP_curr.pos;
SP_des_vel = inbus.SP_des.vel;
SP_des_pos = inbus.SP_des.pos;
WP_idx = inbus.WP_all.idx + 1;
WP_list = inbus.WP_all.list;
std_dev = inbus.std_dev;
current_spline = inbus.current_spline;

children = get(gca, 'children');
delete(children(1:13));

P0 = current_spline(1,:);
P1 = current_spline(2,:);
P2 = current_spline(3,:);
P3 = current_spline(4,:);

% flown track + ground track
plot3(drone_pos(1),drone_pos(2),drone_pos(3),'m.','MarkerSize',7); %1
plot3(drone_pos(1),drone_pos(2),0,'k.','MarkerSize',5); %2

% all WPts + ori
% quiver3 (WP_list(:,1),WP_list(:,2),WP_list(:,3),cos(WP_list(:,4)),sin(WP_list(:,4)),zeros(4,1),0,'c','MaxHeadSize',1,'LineWidth',2); %3
for i = 1:4
    if i == WP_idx
        continue
    end
    plot3(WP_list(i,1)+[0 cos(WP_list(i,4))],WP_list(i,2)+[0 sin(WP_list(i,4))],WP_list(i,3)+[0 0],'c+-','LineWidth',2,'MarkerIndices',2); %3
end

% WP average pos+ori
% quiver3(P2(1),P2(2),P2(3),cos(P2(4)),sin(P2(4)),0,0,'r','MaxHeadSize',1,'LineWidth',2); %4
plot3(WP_list(WP_idx,1)+[0 cos(WP_list(WP_idx,4))],WP_list(WP_idx,2)+[0 sin(WP_list(WP_idx,4))],WP_list(WP_idx,3)+[0 0],'r+-','LineWidth',2,'MarkerIndices',2); %3

% spline
d = (0:0.05:1)';
% u = ones(1,3);
% spline_pos_quad = (1-d)*u.*((1-d)*P0+d*P1)+d*u.*((1-d)*P1 + d*P2);
spline_pos_cubic = (1-d).^3*P0 + 3*(1-d).^2.*d*P1 + 3*(1-d).*d.^2*P2 + d.^3*P3;
plot3(spline_pos_cubic(:,1),spline_pos_cubic(:,2),spline_pos_cubic(:,3),':','Color',[1,0.7,0],'LineWidth',2); %5

% drone pos+vel
plot3(drone_pos(1)+[0 drone_vel(1)],drone_pos(2)+[0 drone_vel(2)],drone_pos(3)+[0 drone_vel(3)],'kx-','LineWidth',1.2,'MarkerIndices',1,'MarkerSize',10); %6

% drone ori
gRb = eul2rotm([drone_ori(3),drone_ori(2),drone_ori(1)]);
length = 1;
x_bebop = gRb*[length;0;0];
y_bebop = gRb*[0;length;0];
z_bebop = gRb*[0;0;length];
plot3(drone_pos(1)+x_bebop(1)*[0.2 1],drone_pos(2)+x_bebop(2)*[0.2 1],drone_pos(3)+x_bebop(3)*[0.2 1],'r--','LineWidth',1.5); %7
plot3(drone_pos(1)+y_bebop(1)*[0.2 1],drone_pos(2)+y_bebop(2)*[0.2 1],drone_pos(3)+y_bebop(3)*[0.2 1],'g--','LineWidth',1.5); %8
plot3(drone_pos(1)+z_bebop(1)*[0.2 1],drone_pos(2)+z_bebop(2)*[0.2 1],drone_pos(3)+z_bebop(3)*[0.2 1],'b--','LineWidth',1.5); %9

% nav pt pos+vel, (yaw)
plot3(SP_des_pos(1)+[0 SP_des_vel(1)],SP_des_pos(2)+[0 SP_des_vel(2)],SP_des_pos(3)+[0 SP_des_vel(3)],'b+-','LineWidth',1.2,'MarkerIndices',1,'MarkerSize',10); %10
% plot3(WP_pos(1)+[0 0.5*cos(WP_yaw)],WP_pos(2)+[0 0.5*sin(WP_yaw)],WP_pos(3)+[0 0],'r-','LineWidth',1)

% WP current pos + ori
if isequal(WP_curr_eul, zeros(1,3)) || isequal(WP_curr_eul, zeros(3,1))
    % no gate info
    WP_curr_pos = [0,0,-100]';
    x_gate = WP_curr_eul;
else   
    gate_rot = eul2rotm(WP_curr_eul');
    x_gate = gate_rot(:,1);
end
% quiver3(gate_pos_global(1),gate_pos_global(2),gate_pos_global(3),x_gate(1),x_gate(2),x_gate(3),0,'b','MaxHeadSize',1,'LineWidth',2); %11
plot3(WP_curr_pos(1)+[0 x_gate(1)],WP_curr_pos(2)+[0 x_gate(2)],WP_curr_pos(3)+[0 x_gate(3)],'b+-','LineWidth',2,'MarkerIndices',2); %3

% WP std dev
std_dev = std_dev*std_dev_factor;
r=linspace(-WP_list(WP_idx,4)+pi/2,-WP_list(WP_idx,4)+5/2*pi,4*4+1)';
angle_std_dev_length=0.6;
angle_std_dev_draw = [WP_list(WP_idx,1:3);
    WP_list(WP_idx,1:3)+angle_std_dev_length*[cos(WP_list(WP_idx,4)+std_dev(4)), sin(WP_list(WP_idx,4)+std_dev(4)), 0];
    WP_list(WP_idx,1:3);
    WP_list(WP_idx,1:3)+angle_std_dev_length*[cos(WP_list(WP_idx,4)-std_dev(4)), sin(WP_list(WP_idx,4)-std_dev(4)), 0];
    WP_list(WP_idx,1:3);
    WP_list(WP_idx,1)+std_dev(1)*sin(r), WP_list(WP_idx,2)+std_dev(2)*cos(r), WP_list(WP_idx,3)+0*r];
d = angle_std_dev_draw;
plot3(d(:,1),d(:,2),d(:,3),':r','LineWidth',1); %12
% [ellx,elly,ellz] = ellipsoid(P2(1),P2(2),P2(3),3*std_dev(1),3*std_dev(2),3*std_dev(3),20);
% surf(ellx,elly,ellz,ellz,'FaceAlpha',0.5)

% legend
% legend(legends(1:12),'flown track','ground track','inactive WP +ori','active WP +ori','spline','drone pos+vel','drone x','drone y','drone z','des pos+vel','measured WP','std dev (x,y,th)','Location','eastoutside')

== matlab function Bebop5_like3_but_dist_toward_end/Guidance/select_WP ==
  data: WP_average output; WP_list input; WP_last output; WP_idx input
function [WP_average, WP_last] = select_WP(WP_list, WP_idx)
    WP_average=zeros(1,4);
    WP_last=zeros(1,4);
    
    WP_average = WP_list(WP_idx+1,:);
    if WP_idx > 0
        WP_last = WP_list(WP_idx,:);
    else
        WP_last = WP_list(end,:);
    end
end

== matlab function Bebop5_like3_but_dist_toward_end/Guidance/create_spline ==
  data: WP_average input; current_spline output size=[4,3]; WP_last input; std_dev input; SP_pos input; d_transformed output
function [current_spline, d_transformed] = create_spline(WP_average, WP_last, std_dev, SP_pos)
% current_spline = zeros(3,3); %4x3
std_dev_factor = 1.0;
std_dev_switch = std_dev_factor/5;

std_dev_radius = std_dev_factor*max(std_dev.*[1;1;1;1/(30*pi/180)]);
std_dev_radius = min(1,std_dev_radius);
HFOV = 1.05*320/200;

WP1 = WP_last(1:4);
WP2 = WP_average(1:4);

offset1 = (std_dev_radius+0.7)/sin(HFOV/2);
if std_dev_radius > std_dev_switch
    WP2(1:3) = WP2(1:3) - offset1*[cos(WP2(4)) sin(WP2(4)) 0];
end

%% position cubic spline real cubic
% % B(d) = (1-d)^3*P0 + 3(1-d)^2*d*P1 + 3(1-d)*d^2*P2 + d^3*P3
% % B'(d) = 3(1-d)^2(P1-P0) + 6*(1-d)*d*(P2-P1) + 3d^2(P3-P2)
% 
% % B(0) = P0
% % B(1) = P3
% 
% P0 = WP1(1:3);
% P3 = WP2(1:3);
% hdg0 = WP1(4);
% hdg3 = WP2(4);
% 
% m=1;
% P1 = [P0(1)+m*cos(hdg0), P0(2)+m*sin(hdg0), P3(3)];
% 
% % n=3;
% % P2 = P3 - [n*cos(hdg3), n*sin(hdg3), 0              ];
% 
% offset2 = (std_dev_factor+0.7)/sin(HFOV/2*0.999);
% P2 = WP_average(1:3) - (offset2+1*(offset2-offset1))*[cos(WP2(4)) sin(WP2(4)) 0];
%      
% current_spline = [P0; P1; P2; P3];

%% position cubic spline through same point
% B(d) = (1-d)^3*P0 + 3(1-d)^2*d*P1 + 3(1-d)*d^2*P2 + d^3*P3
% B'(d) = 3(1-d)^2(P1-P0) + 6*(1-d)*d*(P2-P1) + 3d^2(P3-P2)

% B(0) = P0
% B(1) = P3

P0 = WP1(1:3);
P3 = WP2(1:3);
hdg0 = WP1(4);
hdg3 = WP2(4);

m=1;
P1 = [P0(1)+m*cos(hdg0), P0(2)+m*sin(hdg0), P3(3)];

% n=3;
% P2 = P3 - [n*cos(hdg3), n*sin(hdg3), 0              ];


% Ad^3+Bd^2+Cd+D = 0
x0 = P0(1);
x1 = P1(1);
x3 = P3(1);
y0 = P0(2);
y1 = P1(2);
y3 = P3(2);

xs = SP_pos(1);
ys = SP_pos(2);

if mod(floor((hdg3+pi/4)/(pi/2)),2) % cos/sin
    A = -x0+3*x1-3*x3-cos(hdg3)/sin(hdg3)*(-y0+3*y1-3*y3+y3)+x3;
    B = 3*x0-6*x1+3*x3-cos(hdg3)/sin(hdg3)*(3*y0-6*y1+3*y3);
    C = -3*x0+3*x1-cos(hdg3)/sin(hdg3)*(-3*y0+3*y1);
    D = x0 - cos(hdg3)/sin(hdg3)*(-ys+y0) - xs;
else % sin/cos
    A = -y0+3*y1-3*y3-sin(hdg3)/cos(hdg3)*(-x0+3*x1-3*x3+x3)+y3;
    B = 3*y0-6*y1+3*y3-sin(hdg3)/cos(hdg3)*(3*x0-6*x1+3*x3);
    C = -3*y0+3*y1-sin(hdg3)/cos(hdg3)*(-3*x0+3*x1);
    D = y0 - sin(hdg3)/cos(hdg3)*(-xs+x0) - ys;
end

p = (9*A*C-3*B*B)/(9*A*A);
q = (2*B*B*B-9*A*B*C+27*A*A*D)/(27*A*A*A);
delta = (q/2)*(q/2) + (p/3)*(p/3)*(p/3);

d1 = 0+0i;
d2 = 0+0i;
d3 = 0+0i;
if delta > 0
    u = (-q/2+sqrt(delta))^(1/3);
    v = (-q/2-sqrt(delta))^(1/3);
    d1 = u+v-B/3/A;
    d2 = (u+v)/2 - B/3/A + (u-v)/2*1i*sqrt(3);
    d3 = (u+v)/2 - B/3/A - (u-v)/2*1i*sqrt(3);
elseif delta == 0 && p == 0
    d1 = -B/3/A;
elseif delta == 0 && p ~= 0
    d1 = 3*q/p - B/3/A;
    d2 = -3*q/2/p - B/3/A;
elseif delta < 0
    d1 = -sqrt(-4/3*p)*cos(1/3*acos(-q/2*sqrt(-27/p^3))+pi/3)-B/3/A;
    d2 =  sqrt(-4/3*p)*cos(1/3*acos(-q/2*sqrt(-27/p^3))+ 0/3)-B/3/A;
    d3 = -sqrt(-4/3*p)*cos(1/3*acos(-q/2*sqrt(-27/p^3))-pi/3)-B/3/A;
end

ds = real([d1,d2,d3]);
[~,i]=min(abs(ds-0.5));
d = ds(i);

if mod(floor((hdg3+pi/4)/(pi/2)),2) % cos/sin
    n = (-ys+y0*(1-d)^3+3*d*(1-d)^2*y1+3*d^2*(1-d)*y3+d^3*y3)/(3*d^2*(1-d)*sin(hdg3));
%     n1 = (-ys+y0*(1-d1)^3+3*d1*(1-d1)^2*y1+3*d1^2*(1-d1)*y3+d1^3*y3)/(3*d1^2*(1-d1)*sin(hdg3));
%     n2 = (-ys+y0*(1-d2)^3+3*d2*(1-d2)^2*y1+3*d2^2*(1-d2)*y3+d2^3*y3)/(3*d2^2*(1-d2)*sin(hdg3));
%     n3 = (-ys+y0*(1-d3)^3+3*d3*(1-d3)^2*y1+3*d3^2*(1-d3)*y3+d3^3*y3)/(3*d3^2*(1-d3)*sin(hdg3));
else % sin/cos   
    n = (-xs+x0*(1-d)^3+3*d*(1-d)^2*x1+3*d^2*(1-d)*x3+d^3*x3)/(3*d^2*(1-d)*cos(hdg3));
%     n1 = (-xs+x0*(1-d1)^3+3*d1*(1-d1)^2*x1+3*d1^2*(1-d1)*x3+d1^3*x3)/(3*d1^2*(1-d1)*cos(hdg3));
%     n2 = (-xs+x0*(1-d2)^3+3*d2*(1-d2)^2*x1+3*d2^2*(1-d2)*x3+d2^3*x3)/(3*d2^2*(1-d2)*cos(hdg3));
%     n3 = (-xs+x0*(1-d3)^3+3*d3*(1-d3)^2*x1+3*d3^2*(1-d3)*x3+d3^3*x3)/(3*d3^2*(1-d3)*cos(hdg3));
end

if abs(n) > 10 
    n = 0.001;
end

P2 = P3 - n*[cos(WP2(4)) sin(WP2(4)) 0];
     
current_spline = [P0; P1; P2; P3];
d_transformed = d;
end

== matlab function Bebop5_like3_but_dist_toward_end/Navigation/set position/calculate rest distance ==
  data: d input; spline_new input; d_new output; spline_old input; WP_this input; dist_new output; dist_old output
function [d_new, dist_new, dist_old] = calculate_factor(d, spline_new,spline_old, WP_this)

    P0_old = spline_old(1,:);
    P1_old = spline_old(2,:);
    P2_old = spline_old(3,:);
    P3_old = spline_old(4,:);
    P0_new = spline_new(1,:);
    P1_new = spline_new(2,:);
    P2_new = spline_new(3,:);
    P3_new = spline_new(4,:);
    
    if ~isequal(P0_old,P0_new)
        d_new = d;
        dist_new = 0;
        dist_old = 0;
        return
    end
    
    dx0_new=P1_new(1)-P0_new(1);
    dx1_new=P2_new(1)-P1_new(1);
    dx2_new=P3_new(1)-P2_new(1);
    dy0_new=P1_new(2)-P0_new(2);
    dy1_new=P2_new(2)-P1_new(2);
    dy2_new=P3_new(2)-P2_new(2);
    dx0_old=P1_old(1)-P0_old(1);
    dx1_old=P2_old(1)-P1_old(1);
    dx2_old=P3_old(1)-P2_old(1);
    dy0_old=P1_old(2)-P0_old(2);
    dy1_old=P2_old(2)-P1_old(2);
    dy2_old=P3_old(2)-P2_old(2);
    
    fun_new = @(d_s) 3*sqrt((1-d_s).^4*(dx0_new^2+dy0_new^2)+4*d_s.^2.*(1-d_s).^2*(dx1_new^2+dy1_new^2)+d_s.^4*(dx2_new^2+dy2_new^2)+4*d_s.*(1-d_s).^3*(dx0_new*dx1_new+dy0_new*dy1_new)+2*d_s.^2.*(1-d_s).^2*(dx0_new*dx2_new+dy0_new*dy2_new)+4*d_s.^3.*(1-d_s)*(dx1_new*dx2_new+dy1_new*dy2_new));
    fun_old = @(d_s) 3*sqrt((1-d_s).^4*(dx0_old^2+dy0_old^2)+4*d_s.^2.*(1-d_s).^2*(dx1_old^2+dy1_old^2)+d_s.^4*(dx2_old^2+dy2_old^2)+4*d_s.*(1-d_s).^3*(dx0_old*dx1_old+dy0_old*dy1_old)+2*d_s.^2.*(1-d_s).^2*(dx0_old*dx2_old+dy0_old*dy2_old)+4*d_s.^3.*(1-d_s)*(dx1_old*dx2_old+dy1_old*dy2_old));
%     fnc=3*sqrt((1-d_s)^4*(dx0^2+dy0^2)+4*d_s^2*(1-d_s)^2*(dx1^2+dy1^2)+d_s^4*(dx2^2+dy2^2)+4*d_s*(1-d_s)^3*(dx0*dx1+dy0*dy1)+2*d_s^2*(1-d_s)^2*(dx0*dx2+dy0*dy2)+4*d_s^3*(1-d_s)*(dx1*dx2+dy1*dy2));
%     fnc_num = subs(fnc,d_s,d_num);
    
    d_num = 1:-0.01:d; %linspace(d,1,100);
    dist_new = 0.01*sum(fun_new(d_num));
    dist_old = 0.01*sum(fun_old(d_num));
    
    dist_new = dist_new + norm(P3_new-WP_this(1:3));
    dist_old = dist_old + norm(P3_old-WP_this(1:3));
    
    d_new = d +(dist_new-dist_old)/fun_new(d);
%     dist_new = integral(fun_new,0,d);
%     dist_old = integral(fun_old,0,d);
    
%     d_new = d + (dist_old-dist_new)/fun_new(d);
